simulink model "sf_eventfcn"  (Simulink 7.6)
settings: Solver=ode45  StartTime=0.0  StopTime=30  MaxStep=1  RelTol=1e-3
settings Model: Creator=The MathWorks Inc.  CovMetricSettings=dcmtr  ExtModeAutoUpdateStatusClock=off
settings DataIOCC: SignalLoggingName=sigsOut
settings OptimizationCC: BooleanDataType=off  InlineInvariantSignals=on  InitFltsAndDblsToZero=on  EfficientMapNaN2IntZero=off
settings DebuggingCC: SaveWithParameterizedLinksMsg=none  SignalResolutionControl=TryResolveAllWithWarning  SolverPrmCheckMsg=none  MultiTaskDSMMsg=warning  MultiTaskCondExecSysMsg=none  StrictBusMsg=None
settings HardwareCC: TargetUnknown=on
settings SFSimCC: SimParseCustomCode=off
settings RTWCC: IncludeERTFirstTime=on
settings GRTTargetCC: TargetFcnLib=ansi_tfl_tmw.mat

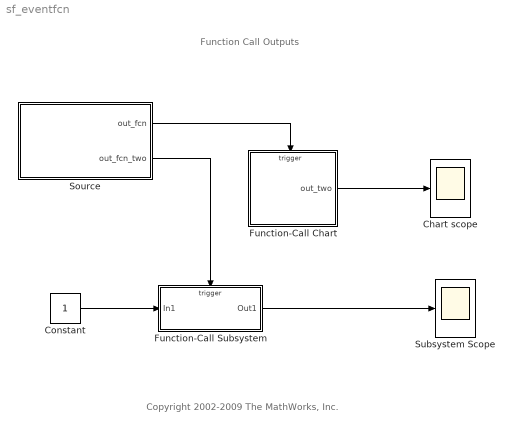
== system sf_eventfcn ==
  note: Function Call Outputs
  note: Copyright 2002-2009 The MathWorks, Inc.
  Chart scope : Scope
      settings: TimeRange=30  YMin=0  YMax=1
  Constant : Constant
  Function-Call Subsystem : Subsystem  TreatAsAtomicUnit=on
  Function-Call Chart : Stateflow chart  TreatAsAtomicUnit=on
  Source : Stateflow chart  TreatAsAtomicUnit=on
  Subsystem Scope : Scope
      settings: TimeRange=30  YMin=0  YMax=2
  wires:
  Source/2(out_fcn_two) -> Function-Call Subsystem/Trigger
  Source/1(out_fcn) -> Function-Call Chart/Trigger
  Function-Call Chart/1(out_two) -> Chart scope/1
  Constant/1 -> Function-Call Subsystem/1(In1)
  Function-Call Subsystem/1(Out1) -> Subsystem Scope/1

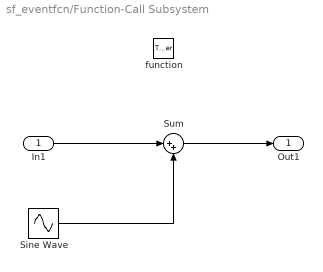
== system sf_eventfcn/Function-Call Subsystem ==
  In1 : Inport
  function : TriggerPort  TriggerType=function-call  ZeroCross=off
  Sine Wave : Sin
  Sum : Sum  Inputs=|++  SaturateOnIntegerOverflow=on  InputSameDT=on  OutDataTypeStr=Inherit: Same as first input
  Out1 : Outport
  wires:
  In1/1 -> Sum/1
  Sum/1 -> Out1/1
  Sine Wave/1 -> Sum/2

== stateflow chart Source ==
  state One [parallel]
    settings: executionOrder=1
    state A
    A -> A : after(3,wakeup)/out_fcn;
  state Two [parallel]
    settings: executionOrder=2
    state B
    (default) -> B
    B -> B : after(2,wakeup)/out_fcn_two;
  (default) -> A
  events: out_fcn output FUNCTION_CALL_EVENT; out_fcn_two output FUNCTION_CALL_EVENT

== stateflow chart Function-Call Chart ==
  state A
    en:out_two=0;
  state B
    en:out_two=1;
  (default) -> A
  A -> B
  B -> A
  data: out_two output double
  events: event input FUNCTION_CALL_EVENT
